simulink model "AADM_xplane10"  (R2018b)
settings: Solver=FixedStepAuto  StartTime=0.0  StopTime=10.0  RelTol=1e-3
undefined symbols (not defined in the file): selecting_parameters
settings Model: Creator=Daniele Nava  LastModifiedBy=Daniele Nava

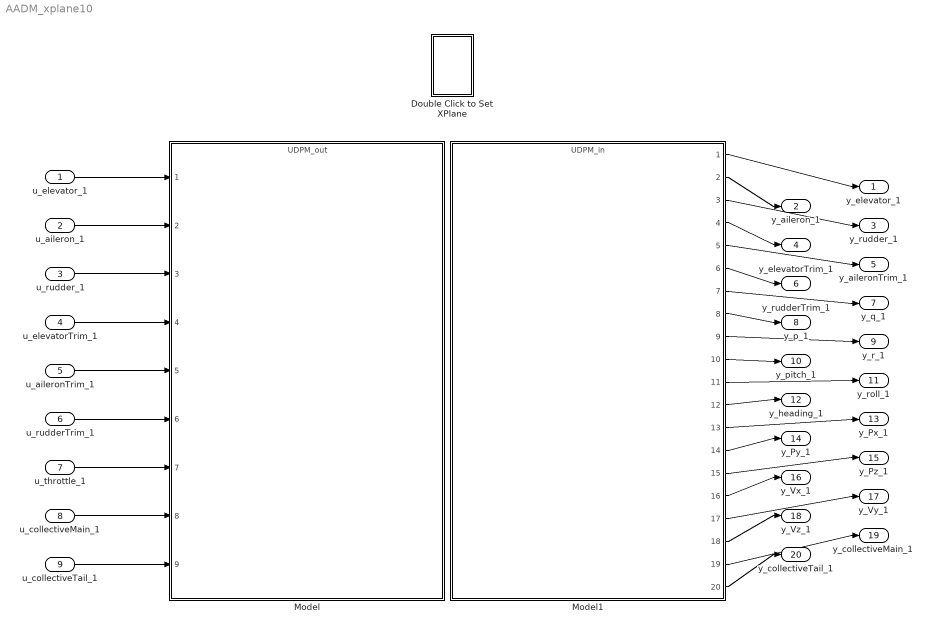
== system AADM_xplane10 ==
  u_elevator_1 : Inport
  u_aileron_1 : Inport  Port=2
  u_rudder_1 : Inport  Port=3
  u_elevatorTrim_1 : Inport  Port=4
  u_aileronTrim_1 : Inport  Port=5
  u_rudderTrim_1 : Inport  Port=6
  u_throttle_1 : Inport  Port=7
  u_collectiveMain_1 : Inport  Port=8
  u_collectiveTail_1 : Inport  Port=9
  Double Click to Set XPlane : Subsystem  LoadFcn=selecting_parameters()
      settings: OpenFcn=selecting_parameters()
  Model : ModelReference  ModelNameDialog=UDPM_out.slx  SimulationMode=Normal  ModelReferenceVersion=1.7
  Model1 : ModelReference  ModelNameDialog=UDPM_in.slx  SimulationMode=Normal  ModelReferenceVersion=1.11
  y_elevator_1 : Outport
  y_aileron_1 : Outport  Port=2
  y_rudder_1 : Outport  Port=3
  y_elevatorTrim_1 : Outport  Port=4
  y_aileronTrim_1 : Outport  Port=5
  y_rudderTrim_1 : Outport  Port=6
  y_q_1 : Outport  Port=7
  y_p_1 : Outport  Port=8
  y_r_1 : Outport  Port=9
  y_pitch_1 : Outport  Port=10
  y_roll_1 : Outport  Port=11
  y_heading_1 : Outport  Port=12
  y_Px_1 : Outport  Port=13
  y_Py_1 : Outport  Port=14
  y_Pz_1 : Outport  Port=15
  y_Vx_1 : Outport  Port=16
  y_Vy_1 : Outport  Port=17
  y_Vz_1 : Outport  Port=18
  y_collectiveMain_1 : Outport  Port=19
  y_collectiveTail_1 : Outport  Port=20
  wires:
  u_rudder_1/1 -> Model/3
  u_aileronTrim_1/1 -> Model/5
  u_throttle_1/1 -> Model/7
  u_rudderTrim_1/1 -> Model/6
  u_collectiveMain_1/1 -> Model/8
  u_collectiveTail_1/1 -> Model/9
  u_elevator_1/1 -> Model/1
  u_aileron_1/1 -> Model/2
  u_elevatorTrim_1/1 -> Model/4
  Model1/1 -> y_elevator_1/1
  Model1/2 -> y_aileron_1/1
  Model1/3 -> y_rudder_1/1
  Model1/4 -> y_elevatorTrim_1/1
  Model1/5 -> y_aileronTrim_1/1
  Model1/6 -> y_rudderTrim_1/1
  Model1/7 -> y_q_1/1
  Model1/8 -> y_p_1/1
  Model1/9 -> y_r_1/1
  Model1/10 -> y_pitch_1/1
  Model1/11 -> y_roll_1/1
  Model1/12 -> y_heading_1/1
  Model1/13 -> y_Px_1/1
  Model1/14 -> y_Py_1/1
  Model1/15 -> y_Pz_1/1
  Model1/16 -> y_Vx_1/1
  Model1/17 -> y_Vy_1/1
  Model1/18 -> y_Vz_1/1
  Model1/20 -> y_collectiveTail_1/1
  Model1/19 -> y_collectiveMain_1/1

== system AADM_xplane10/Double Click to Set XPlane ==
